simulink subsystem "Timer"  (R2020a)
settings: Solver=VariableStepAuto  StartTime=0.0  StopTime=10.0  RelTol=1e-3
settings Model: Creator=zinoex  LastModifiedBy=zinoex

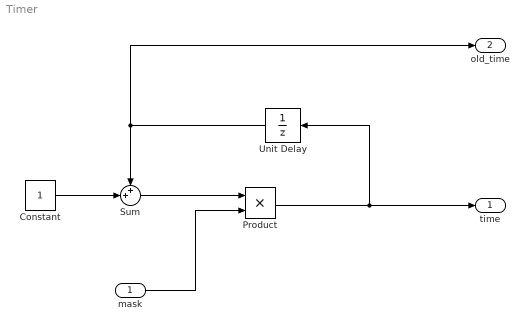
== system Timer ==
  mask : Inport
  Constant : Constant
  Product : Product
  Sum : Sum  Inputs=++|
  Unit Delay : UnitDelay  SampleTime=-1  HasFrameUpgradeWarning=on
  time : Outport
  old_time : Outport  Port=2
  wires:
  Unit Delay/1 -> old_time/1, Sum/1
  Product/1 -> time/1, Unit Delay/1
  Constant/1 -> Sum/2
  Sum/1 -> Product/1
  mask/1 -> Product/2
